simulink model "Digital_Adaptive_RBF_Control_For_Continuous_System"  (R2023a)
settings: Solver=VariableStepAuto  StartTime=0.0  StopTime=10.0  RelTol=1e-3
settings Model: Creator=ACCENT  LastModifiedBy=ACCENT

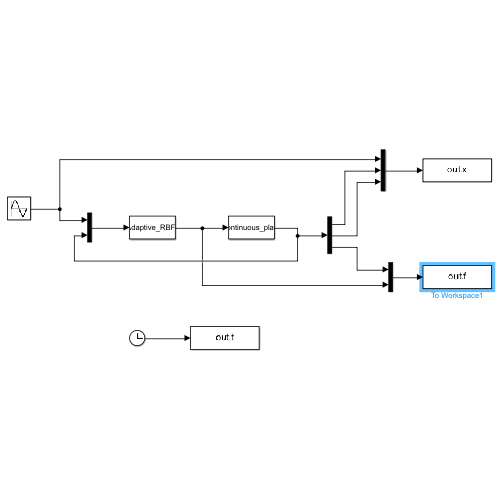
[thumbnail: Simulink's stored preview of the top-level diagram]
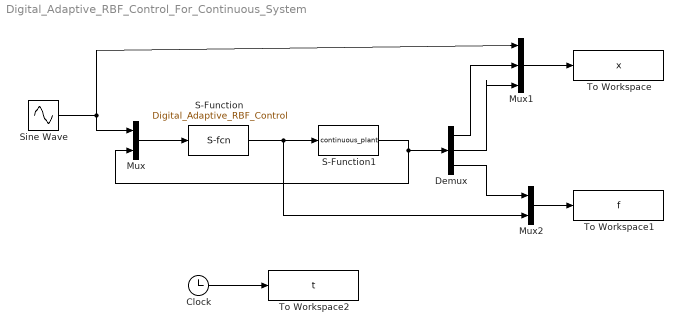
== system Digital_Adaptive_RBF_Control_For_Continuous_System ==
  Clock : Clock
  Demux : Demux  Outputs=3
  Mux : Mux  Inputs=2
  Mux1 : Mux  Inputs=3
  Mux2 : Mux  Inputs=2
  S-Function : S-Function  FunctionName=Digital_Adaptive_RBF_Control  SFunctionDeploymentMode=off  EnableBusSupport=off
  S-Function1 : S-Function  FunctionName=continuous_plant  SFunctionDeploymentMode=off  EnableBusSupport=off
  Sine Wave : Sin  SampleTime=0
  To Workspace : ToWorkspace  VariableName=x  SampleTime=-1
  To Workspace1 : ToWorkspace  VariableName=f  SampleTime=-1
  To Workspace2 : ToWorkspace  VariableName=t  SampleTime=-1
  wires:
  Mux2/1 -> To Workspace1/1
  Clock/1 -> To Workspace2/1
  Mux/1 -> S-Function/1
  S-Function/1 -> Mux2/2, S-Function1/1
  S-Function1/1 -> Mux/2, Demux/1
  Demux/3 -> Mux2/1
  Mux1/1 -> To Workspace/1
  Demux/2 -> Mux1/3
  Demux/1 -> Mux1/2
  Sine Wave/1 -> Mux/1, Mux1/1
